simulink model "Block_test"  (R2018a)
settings: Solver=VariableStepAuto  StartTime=0.0  StopTime=10.0  RelTol=1e-3
libraries: vrlib x1
settings Model: Creator=WEIDONG  LastModifiedBy=WEIDONG

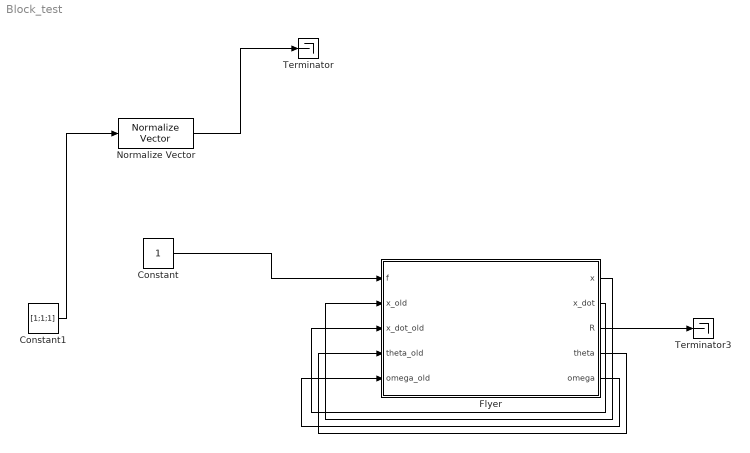
== system Block_test ==
  Constant : Constant
  Constant1 : Constant  Value=[1;1;1]  VectorParams1D=off
  Flyer : MATLAB Function  TreatAsAtomicUnit=on
  Normalize Vector : vrlib/Utilities/Normalize Vector  maxzero=0
      settings: SourceProductName=Simulink 3D Animation  SourceProductBaseCode=VR
  Terminator : Terminator
  Terminator3 : Terminator
  wires:
  Normalize Vector/1 -> Terminator/1
  Constant1/1 -> Normalize Vector/1
  Constant/1 -> Flyer/1(f)
  Flyer/1(x) -> Flyer/2(x_old)
  Flyer/2(x_dot) -> Flyer/3(x_dot_old)
  Flyer/3(R) -> Terminator3/1
  Flyer/4(theta) -> Flyer/4(theta_old)
  Flyer/5(omega) -> Flyer/5(omega_old)

== matlab function Block_test/Flyer ==
  data: f input; x_old input; x_dot_old input; x output; x_dot output; R output; theta output; theta_old input; omega_old input; omega output
function [x,x_dot,R,theta,omega] = fcn(f,x_old,x_dot_old,theta_old,omega_old)
% the block is based on the dynamics of a quadcopter on
% http://andrew.gibiansky.com/blog/physics/quadcopter-dynamics/
    
    %initial states
    %row, pitch and yaw
    theta = zeros(3,1);
    thetadot = zeros(3,1);

    %parameters
    g = [0; 0; -9.8];
    m = 0.5;
    d = [0,0,0.17];

    I_B_B = diag([2.7*10e-3, 2.7*10e-3,5.2*10e-3]);  % Body Inertia
    I_B_P = diag([0, 0,1.5*10e-5]);  % Propeller Inertia

    dt=0.01;%simulation time interval in seconds

    %aerodynamic drag torque
    K_B_d=diag([0.7*10e-4, 0.7*10e-4, 1.4*10e-4]);

    % Compute thrust given current inputs and thrust coefficient.
    %f = [0; 0; 6.41*10^(-6) * input*input];
    prop_speed_sq=f/(6.41*10^(-6));
    % Compute reaction torque, given current inputs, length, drag coefficient, and thrust coefficient.
    T_p = -prop_speed_sq* 1.1 * 10e-7;
    f_vector=[0; 0; f];
    % Compute forces, torques, and accelerations.
    omega = thetadot2omega(thetadot, theta);
    %acceleration in earth frame
    %R = rotation(theta);%rotation matrix from body frame to earth frame
    R=zeros(3,3);
    T = R * f_vector;
    a = g + (1 / m) .* T;
    %omegadot
    t_B_d=-sqrt(sum((omega).^2))*K_B_d*omega;
    tau=cross(d',f_vector)+T_p;%total torque

    omegadot = I_B_B\ (tau + t_B_d - cross(omega, I_B_B * omega+I_B_P*(R*input)));

    % Advance system state
    omega = omega_old + dt .* omegadot;
    %omega=[0;0;0];
    thetadot = omega2thetadot(omega, theta); 
    theta = theta_old + dt * thetadot;
    %x_dot = x_dot_old + a * dt;
    x_dot=[0;0;0];
    x = x_old + dt .* x_dot;
    %x=[0;0;0];
    %SetOutputPortDimensions(s, 2, [3 1]);
end
